simulink model "continousSystemVisualization"  (R2013a)
settings: Solver=ode45  StartTime=0.0  StopTime=10.0  RelTol=1e-3
settings Model: Creator=GCES  LastModifiedBy=GCES

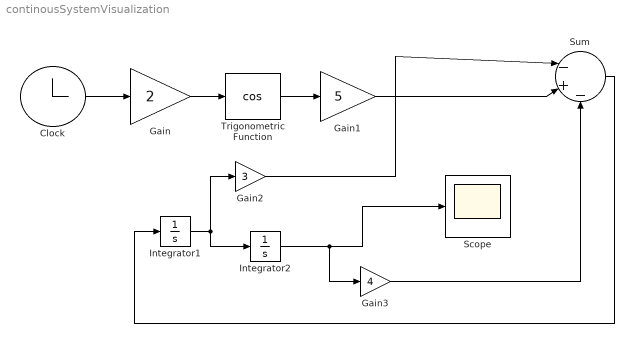
== system continousSystemVisualization ==
  Clock : Clock
  Gain : Gain  Gain=2
  Gain1 : Gain  Gain=5
  Gain2 : Gain  Gain=3
  Gain3 : Gain  Gain=4
  Integrator1 : Integrator
  Integrator2 : Integrator
  Scope : Scope
  Sum : Sum  Inputs=|-+-
  Trigonometric Function : Trigonometry  Operator=cos
  wires:
  Clock/1 -> Gain/1
  Gain/1 -> Trigonometric Function/1
  Trigonometric Function/1 -> Gain1/1
  Gain1/1 -> Sum/2
  Gain2/1 -> Sum/1
  Integrator1/1 -> Gain2/1, Integrator2/1
  Integrator2/1 -> Gain3/1, Scope/1
  Gain3/1 -> Sum/3
  Sum/1 -> Integrator1/1
